simulink model "capsubot_Simulation_comparison_LandC"  (R2019a)
settings: Solver=ode45  StartTime=0.0  StopTime=16  FixedStep=.0001  MaxStep=.001  MinStep=.000001  RelTol=1e-3  EnableMultiTasking=on
values from neighbouring files (symbols this model uses):
  a1 = -a_stoke    [capsubot_dataperfectLuGree.m]
  a_c_desired_backward = [-a_all1' -a_all2']    [capsubot_dataperfectLuGree.m]
  a_u_desired = [a_all2' a_all1' a_all1' a_all2']    [capsubot_dataperfectLuGree.m]
  a_u_desired_backward = [-a_all2' -a_all1' -a_all1' -a_all2']    [capsubot_dataperfectLuGree.m]
  f_sm = data(8)    [capsubot_dataperfectLuGree.m]
  f_sM = 0.49    [capsubot_dataperfectLuGree.m]
  fv_Cap = data(9)    [capsubot_dataperfectLuGree.m]
  fv_IM = data(9)    [capsubot_dataperfectLuGree.m]
  g = 9.8    [capsubot_dataperfectLuGree.m]
  j = 30    [capsubot_dataperfectLuGree.m]
  k1 = 300    [capsubot_dataperfectLuGree.m]
  k2 = 100    [capsubot_dataperfectLuGree.m]
  m = data(2)    [capsubot_dataperfectLuGree.m]
  M = data(1)    [capsubot_dataperfectLuGree.m]
  m1 = data(2)    [capsubot_dataperfectLuGree.m]
  mu = data(3)    [capsubot_dataperfectLuGree.m]
  mu_1 = data(4)    [capsubot_dataperfectLuGree.m]
  mu_m = data(4)    [capsubot_dataperfectLuGree.m]
  sig_cap0 = data(8)    [capsubot_dataperfectLuGree.m]
  sig_cap1 = data(11)    [capsubot_dataperfectLuGree.m]
  sig_IM0 = data(8)    [capsubot_dataperfectLuGree.m]
  sig_IM1 = data(9)    [capsubot_dataperfectLuGree.m]
  tc = zeros(n,2)    [capsubot_dataperfectLuGree.m]
  tu = zeros(n,4)    [capsubot_dataperfectLuGree.m]
  z_cap = data(7)    [capsubot_dataperfectLuGree.m]
  z_IM = data(9)    [capsubot_dataperfectLuGree.m]
undefined symbols (not defined in the file or in its folder): profile, time_sim_individual_cum
libraries: fuzblock x2
(part 1 of 3)
settings Model: Creator=ERAS  LastModifiedBy=moham911
settings SolverCC: InitialStep=.001
settings DataIOCC: SaveFormat=Array  ReturnWorkspaceOutputs=off
settings OptimizationCC: ExpressionDepthLimit=2147483647  LifeSpan=inf
settings DebuggingCC: UnderspecifiedInitializationDetection=Classic  MergeDetectMultiDrivingBlocksExec=none  SolverPrmCheckMsg=warning  FcnCallInpInsideContextMsg=warning  StateNameClashWarn=warning  SFUnexpectedBacktrackingDiag=warning  SFNoUnconditionalDefaultTransitionDiag=warning  SFExecutionAtInitializationDiag=none  ArithmeticOperatorsInVariantConditions=warning
settings HardwareCC: ProdBitPerPointer=32  ProdBitPerSizeT=32  ProdBitPerPtrDiffT=32  ProdLargestAtomicFloat=None  ProdIntDivRoundTo=Undefined  ProdEndianess=Unspecified  ProdWordSize=32  ProdHWDeviceType=32-bit Generic
settings ModelReferenceCC: PropagateSignalLabelsOutOfModel=off
settings SFSimCC: SimUseLocalCustomCode=off
settings RTWCC: RTWUseLocalCustomCode=off
settings CodeAppCC: StateflowObjectComments=on
settings GRTTargetCC: TargetLangStandard=C89/C90 (ANSI)  GeneratePreprocessorConditionals=Disable all  CombineOutputUpdateFcns=off  GRTInterface=on
settings ConfigComp: CovMetricSettings=dw  CovHtmlReporting=on  CovSaveCumulativeToWorkspaceVar=on  CovSaveSingleToWorkspaceVar=on  CovExternalEMLEnable=off

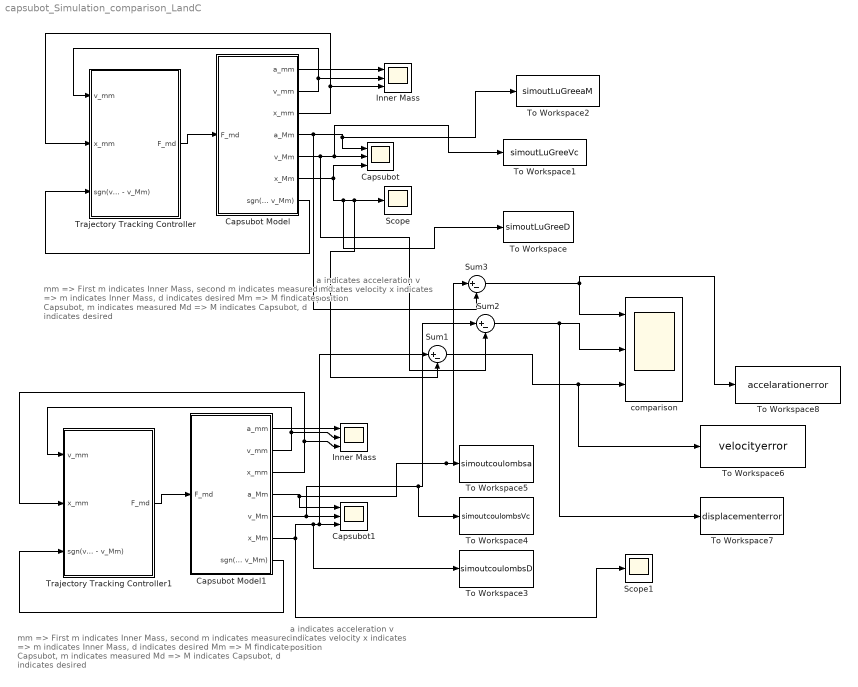
== system capsubot_Simulation_comparison_LandC ==
  note: a indicates acceleration
      | v indicates velocity
      | x indicates position
  note: mm => First m indicates Inner Mass, second m indicates measured
      | md => m indicates Inner Mass, d indicates desired
      | Mm => M findicates Capsubot, m indicates measured
      | Md => M indicates Capsubot, d indicates desired
  note: mm => First m indicates Inner Mass, second m indicates measured
      | md => m indicates Inner Mass, d indicates desired
      | Mm => M findicates Capsubot, m indicates measured
      | Md => M indicates Capsubot, d indicates desired
  note: a indicates acceleration
      | v indicates velocity
      | x indicates position
  " Capsubot Model" : Subsystem
  " Capsubot Model1" : Subsystem
  " Trajectory Tracking Controller" : Subsystem
  " Trajectory Tracking Controller1" : Subsystem
  Capsubot : Scope  NumInputPorts=3
  Capsubot1 : Scope  NumInputPorts=3
  Inner Mass : Scope  NumInputPorts=3
  "Inner Mass " : Scope  NumInputPorts=3
  Scope : Scope
  Scope1 : Scope
  Sum1 : Sum  Inputs=|+-
  Sum2 : Sum  Inputs=|+-
  Sum3 : Sum  Inputs=|+-
  To Workspace : ToWorkspace  VariableName=simoutLuGreeD  SaveFormat=Timeseries  SampleTime=-1
  To Workspace1 : ToWorkspace  VariableName=simoutLuGreeVc  SaveFormat=Timeseries  SampleTime=-1
  To Workspace2 : ToWorkspace  VariableName=simoutLuGreeaM  SaveFormat=Timeseries  SampleTime=-1
  To Workspace3 : ToWorkspace  VariableName=simoutcoulombsD  SaveFormat=Timeseries  SampleTime=-1
  To Workspace4 : ToWorkspace  VariableName=simoutcoulombsVc  SaveFormat=Timeseries  SampleTime=-1
  To Workspace5 : ToWorkspace  VariableName=simoutcoulombsa  SaveFormat=Timeseries  SampleTime=-1
  To Workspace6 : ToWorkspace  VariableName=velocityerror  SaveFormat=Timeseries  SampleTime=-1
  To Workspace7 : ToWorkspace  VariableName=displacementerror  SaveFormat=Timeseries  SampleTime=-1
  To Workspace8 : ToWorkspace  VariableName=accelarationerror  SaveFormat=Timeseries  SampleTime=-1
  "comparison " : Scope  NumInputPorts=3
  wires:
  " Capsubot Model"/2(v_mm) -> " Trajectory Tracking Controller"/1(v_mm), "Inner Mass "/2
  " Capsubot Model"/3(x_mm) -> " Trajectory Tracking Controller"/2(x_mm), "Inner Mass "/3
  " Capsubot Model"/1(a_mm) -> "Inner Mass "/1
  " Capsubot Model"/4(a_Mm) -> Sum3/2, To Workspace2/1, Capsubot/1
  " Capsubot Model"/5(v_Mm) -> Sum2/2, To Workspace1/1, Capsubot/2
  " Capsubot Model"/6(x_Mm) -> Capsubot/3, To Workspace/1, Sum1/2, Scope/1
  " Capsubot Model"/7(sgn(v_mm - v_Mm)) -> " Trajectory Tracking Controller"/3(sgn(v_mm - v_Mm))
  " Trajectory Tracking Controller"/1(F_md) -> " Capsubot Model"/1(F_md)
  " Capsubot Model1"/6(x_Mm) -> Scope1/1, To Workspace3/1, Sum1/1, Capsubot1/3
  " Capsubot Model1"/2(v_mm) -> Inner Mass/2, " Trajectory Tracking Controller1"/1(v_mm)
  " Capsubot Model1"/3(x_mm) -> " Trajectory Tracking Controller1"/2(x_mm), Inner Mass/3
  " Capsubot Model1"/4(a_Mm) -> Sum3/1, To Workspace5/1, Capsubot1/1
  " Capsubot Model1"/5(v_Mm) -> Capsubot1/2, Sum2/1, To Workspace4/1
  " Capsubot Model1"/1(a_mm) -> Inner Mass/1
  " Capsubot Model1"/7(sgn(v_mm - v_Mm)) -> " Trajectory Tracking Controller1"/3(sgn(v_mm - v_Mm))
  " Trajectory Tracking Controller1"/1(F_md) -> " Capsubot Model1"/1(F_md)
  Sum1/1 -> To Workspace6/1, "comparison "/3
  Sum2/1 -> To Workspace7/1, "comparison "/2
  Sum3/1 -> "comparison "/1, To Workspace8/1

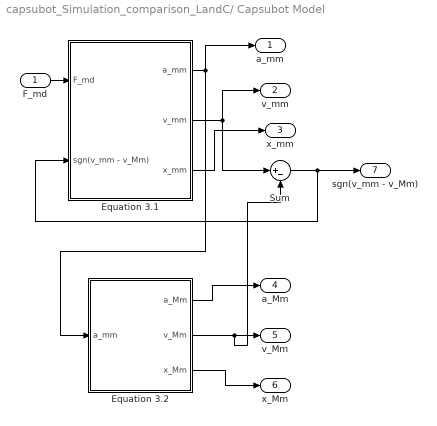
== system capsubot_Simulation_comparison_LandC/ Capsubot Model ==
  F_md : Inport
  Equation 3.1 : Subsystem
  Equation 3.2 : Subsystem
  Sum : Sum  Inputs=|+-
  a_mm : Outport
  v_mm : Outport  Port=2
  x_mm : Outport  Port=3
  a_Mm : Outport  Port=4
  v_Mm : Outport  Port=5
  x_Mm : Outport  Port=6
  sgn(v_mm - v_Mm) : Outport  Port=7
  wires:
  F_md/1 -> Equation 3.1/1(F_md)
  Equation 3.1/1(a_mm) -> a_mm/1, Equation 3.2/1(a_mm)
  Equation 3.1/2(v_mm) -> v_mm/1, Sum/1
  Equation 3.1/3(x_mm) -> x_mm/1
  Equation 3.2/1(a_Mm) -> a_Mm/1
  Equation 3.2/2(v_Mm) -> Sum/2, v_Mm/1
  Equation 3.2/3(x_Mm) -> x_Mm/1
  Sum/1 -> sgn(v_mm - v_Mm)/1, Equation 3.1/2(sgn(v_mm - v_Mm))

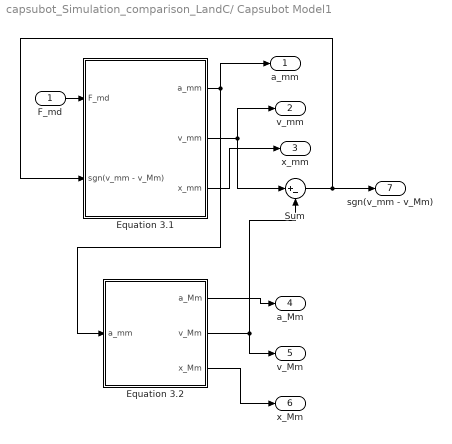
== system capsubot_Simulation_comparison_LandC/ Capsubot Model1 ==
  F_md : Inport
  Equation 3.1 : Subsystem
  Equation 3.2 : Subsystem
  Sum : Sum  Inputs=|+-
  a_mm : Outport
  v_mm : Outport  Port=2
  x_mm : Outport  Port=3
  a_Mm : Outport  Port=4
  v_Mm : Outport  Port=5
  x_Mm : Outport  Port=6
  sgn(v_mm - v_Mm) : Outport  Port=7
  wires:
  F_md/1 -> Equation 3.1/1(F_md)
  Equation 3.1/1(a_mm) -> a_mm/1, Equation 3.2/1(a_mm)
  Equation 3.1/2(v_mm) -> v_mm/1, Sum/1
  Equation 3.1/3(x_mm) -> x_mm/1
  Equation 3.2/1(a_Mm) -> a_Mm/1
  Equation 3.2/2(v_Mm) -> v_Mm/1, Sum/2
  Equation 3.2/3(x_Mm) -> x_Mm/1
  Sum/1 -> sgn(v_mm - v_Mm)/1, Equation 3.1/2(sgn(v_mm - v_Mm))

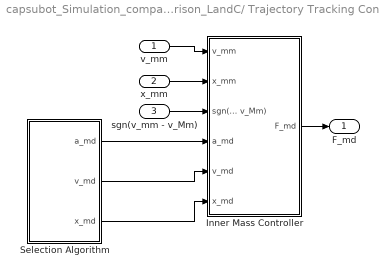
== system capsubot_Simulation_comparison_LandC/ Trajectory Tracking Controller ==
  v_mm : Inport
  x_mm : Inport  Port=2
  sgn(v_mm - v_Mm) : Inport  Port=3
  Inner Mass Controller : Subsystem
  Selection Algorithm : Subsystem
  F_md : Outport
  wires:
  Selection Algorithm/1(a_md) -> Inner Mass Controller/4(a_md)
  Selection Algorithm/3(x_md) -> Inner Mass Controller/6(x_md)
  sgn(v_mm - v_Mm)/1 -> Inner Mass Controller/3(sgn(v_mm - v_Mm))
  Selection Algorithm/2(v_md) -> Inner Mass Controller/5(v_md)
  Inner Mass Controller/1(F_md) -> F_md/1
  v_mm/1 -> Inner Mass Controller/1(v_mm)
  x_mm/1 -> Inner Mass Controller/2(x_mm)

== system capsubot_Simulation_comparison_LandC/ Trajectory Tracking Controller1 ==
  v_mm : Inport
  x_mm : Inport  Port=2
  sgn(v_mm - v_Mm) : Inport  Port=3
  Inner Mass Controller : Subsystem
  Selection Algorithm : Subsystem
  F_md : Outport
  wires:
  Selection Algorithm/1(a_md) -> Inner Mass Controller/4(a_md)
  Selection Algorithm/3(x_md) -> Inner Mass Controller/6(x_md)
  sgn(v_mm - v_Mm)/1 -> Inner Mass Controller/3(sgn(v_mm - v_Mm))
  Selection Algorithm/2(v_md) -> Inner Mass Controller/5(v_md)
  Inner Mass Controller/1(F_md) -> F_md/1
  v_mm/1 -> Inner Mass Controller/1(v_mm)
  x_mm/1 -> Inner Mass Controller/2(x_mm)

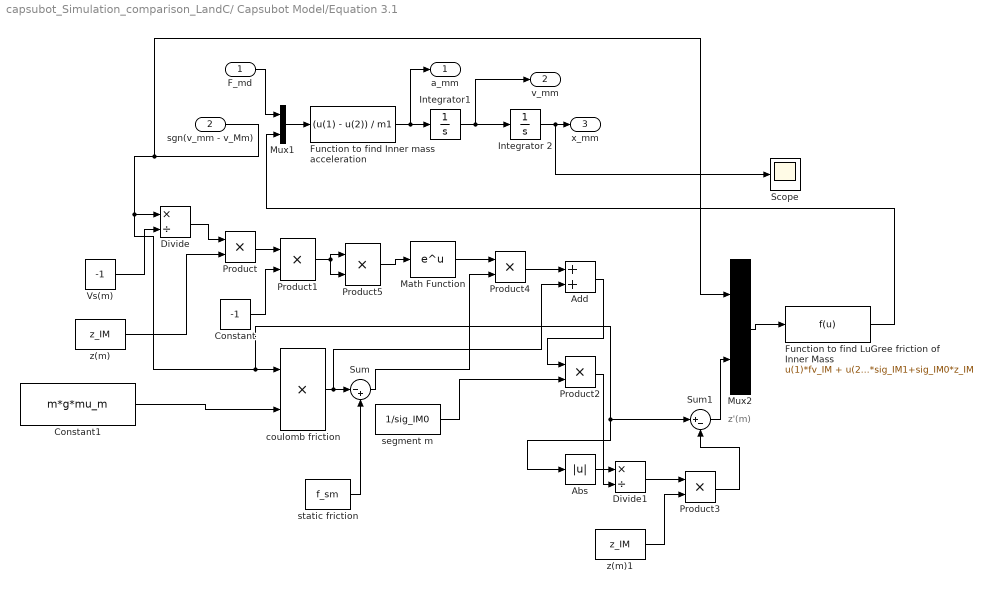
== system capsubot_Simulation_comparison_LandC/ Capsubot Model/Equation 3.1 ==
  note: z'(m)
  F_md : Inport
  sgn(v_mm - v_Mm) : Inport  Port=2
  Abs : Abs
  Add : Sum
  Constant : Constant  Value=-1
  Constant1 : Constant  Value=m*g*mu_m
  Divide : Product  Inputs=*/
  Divide1 : Product  Inputs=*/
  Function to find Inner mass acceleration : Fcn  Expr=(u(1) - u(2)) / m1
  "Function to find LuGree friction of Inner Mass " : Fcn  Expr=u(1)*fv_IM + u(2)*sig_IM1+sig_IM0*z_IM
  Integrator 2 : Integrator  InitialCondition=a1
  Integrator1 : Integrator
  Math Function : Math  SaturateOnIntegerOverflow=on
  Mux1 : Mux  Inputs=2
  Mux2 : Mux  Inputs=2
  Product{,1..5} (6 alike) : Product
  Scope : Scope
  Sum : Sum  Inputs=|-+
  Sum1 : Sum  Inputs=|+-
  Vs(m) : Constant  Value=-1
  "coulomb friction " : Product
  segment m : Constant  Value=1/sig_IM0
  "static friction " : Constant  Value=f_sm
  z(m) : Constant  Value=z_IM
  z(m)1 : Constant  Value=z_IM
  a_mm : Outport
  v_mm : Outport  Port=2
  x_mm : Outport  Port=3
  wires:
  "Function to find LuGree friction of Inner Mass "/1 -> Mux1/2
  Mux1/1 -> Function to find Inner mass acceleration/1
  F_md/1 -> Mux1/1
  Integrator1/1 -> v_mm/1, Integrator 2/1
  Integrator 2/1 -> Scope/1, x_mm/1
  Function to find Inner mass acceleration/1 -> a_mm/1, Integrator1/1
  segment m/1 -> Product2/2
  Product/1 -> Product1/1
  z(m)/1 -> Product/2
  Math Function/1 -> Product4/1
  Product4/1 -> Add/1
  Vs(m)/1 -> Divide/2
  "static friction "/1 -> Sum/2
  Sum/1 -> Product4/2
  Constant1/1 -> "coulomb friction "/2
  Constant/1 -> Product1/2
  Add/1 -> Product2/1
  "coulomb friction "/1 -> Add/2, Sum/1
  Divide/1 -> Product/1
  sgn(v_mm - v_Mm)/1 -> Mux2/1, Abs/1, Sum1/1, "coulomb friction "/1, Divide/1
  Abs/1 -> Divide1/1
  Product2/1 -> Divide1/2
  z(m)1/1 -> Product3/2
  Mux2/1 -> "Function to find LuGree friction of Inner Mass "/1
  Product5/1 -> Math Function/1
  Product1/1 -> Product5/2, Product5/1
  Divide1/1 -> Product3/1
  Product3/1 -> Sum1/2
  Sum1/1 -> Mux2/2

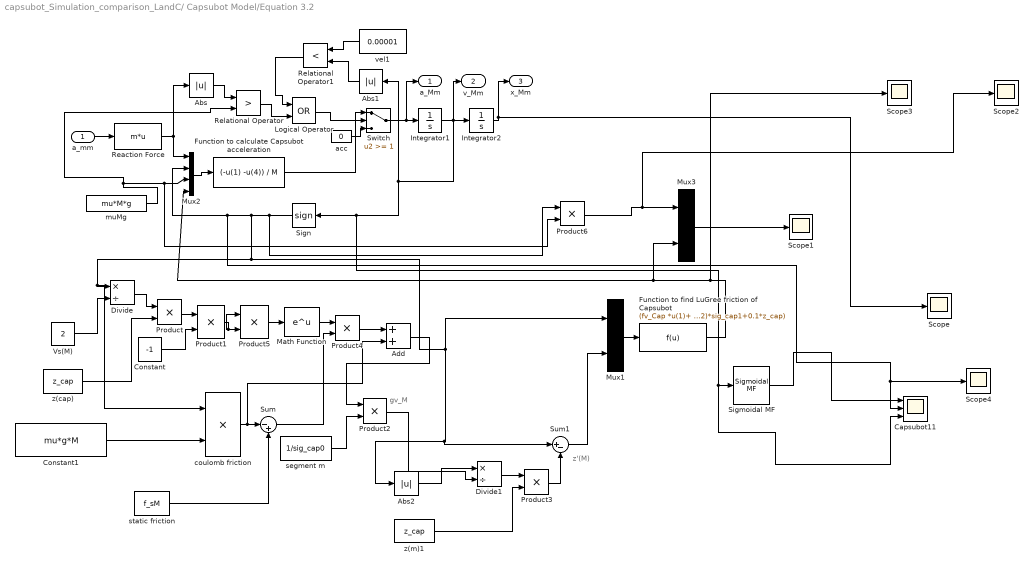
== system capsubot_Simulation_comparison_LandC/ Capsubot Model/Equation 3.2 ==
  note: gv_M
  note: z'(M)
  a_mm : Inport
  Abs : Abs
  Abs1 : Abs
  Abs2 : Abs
  Add : Sum
  Capsubot11 : Scope  NumInputPorts=3
  Constant : Constant  Value=-1
  Constant1 : Constant  Value=mu*g*M
  Divide : Product  Inputs=*/
  Divide1 : Product  Inputs=*/
  Function to calculate Capsubot acceleration : Fcn  Expr=(-u(1) -u(4)) / M
  "Function to find LuGree friction of Capsubot " : Fcn  Expr=(fv_Cap *u(1)+ u(2)*sig_cap1+0.1*z_cap)
  Integrator1 : Integrator
  Integrator2 : Integrator
  Logical Operator : Logic  Operator=OR  AllPortsSameDT=off  OutDataTypeStr=boolean
  Math Function : Math  SaturateOnIntegerOverflow=on
  Mux1 : Mux  Inputs=2
  Mux2 : Mux
  Mux3 : Mux  Inputs=2
  Product{,1..6} (7 alike) : Product
  Reaction Force : Fcn  Expr=m*u
  Relational Operator : RelationalOperator  Operator=>  OutDataTypeStr=boolean  RndMeth=Nearest
  Relational Operator1 : RelationalOperator  Operator=<  OutDataTypeStr=boolean  RndMeth=Nearest
  Scope{,1..4} (5 alike) : Scope
  Sigmoidal MF : fuzblock/Membership  Functions/Sigmoidal MF  a=1/1000  c=0
      settings: SourceProductName=Fuzzy Logic Toolbox  SourceProductBaseCode=FL
  Sign : Signum  ZeroCross=off
  Sum : Sum  Inputs=|-+
  Sum1 : Sum  Inputs=|+-
  Switch : Switch  Threshold=1
  Vs(M) : Constant  Value=2
  acc : Constant  Value=0
  "coulomb friction " : Product
  muMg : Constant  Value=mu*M*g
  segment m : Constant  Value=1/sig_cap0
  "static friction " : Constant  Value=f_sM
  vel1 : Constant  Value=0.00001
  z(cap) : Constant  Value=z_cap
  z(m)1 : Constant  Value=z_cap
  a_Mm : Outport
  v_Mm : Outport  Port=2
  x_Mm : Outport  Port=3
  wires:
  Mux2/1 -> Function to calculate Capsubot acceleration/1
  Abs/1 -> Relational Operator/1
  Function to calculate Capsubot acceleration/1 -> Switch/1
  acc/1 -> Switch/3
  Relational Operator/1 -> Logical Operator/2
  Logical Operator/1 -> Switch/2
  Relational Operator1/1 -> Logical Operator/1
  vel1/1 -> Relational Operator1/1
  Abs1/1 -> Relational Operator1/2
  Sign/1 -> Product6/1, Sum1/1, Abs2/1, Mux1/1, "coulomb friction "/1, Divide/1, Scope4/1, Capsubot11/2, Mux2/2
  muMg/1 -> Relational Operator/2, Product6/2, Mux2/3
  Reaction Force/1 -> Abs/1, Mux2/1
  a_mm/1 -> Reaction Force/1
  Switch/1 -> a_Mm/1, Integrator1/1
  "Function to find LuGree friction of Capsubot "/1 -> Scope3/1, Mux3/2, Mux2/4
  Vs(M)/1 -> Divide/2
  Product4/1 -> Add/1
  Product/1 -> Product1/1
  z(cap)/1 -> Product/2
  segment m/1 -> Product2/2
  Product2/1 -> Divide1/2
  Abs2/1 -> Divide1/1
  Sum/1 -> Product4/2
  "static friction "/1 -> Sum/2
  Constant/1 -> Product1/2
  "coulomb friction "/1 -> Add/2, Sum/1
  Divide/1 -> Product/1
  Integrator1/1 -> Integrator2/1, v_Mm/1, Capsubot11/3, Sigmoidal MF/1, Sign/1, Abs1/1
  Mux1/1 -> "Function to find LuGree friction of Capsubot "/1
  Math Function/1 -> Product4/1
  z(m)1/1 -> Product3/2
  Add/1 -> Product2/1
  Product1/1 -> Product5/1, Product5/2
  Product5/1 -> Math Function/1
  Constant1/1 -> "coulomb friction "/2
  Integrator2/1 -> Scope/1, x_Mm/1
  Divide1/1 -> Product3/1
  Product3/1 -> Sum1/2
  Sum1/1 -> Mux1/2
  Product6/1 -> Scope2/1, Mux3/1
  Mux3/1 -> Scope1/1
  Sigmoidal MF/1 -> Capsubot11/1

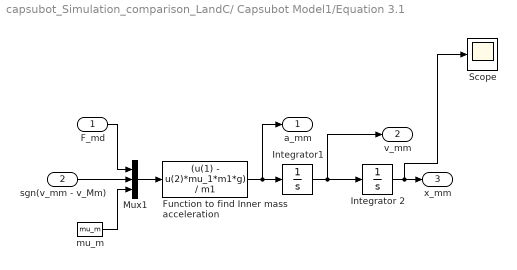
== system capsubot_Simulation_comparison_LandC/ Capsubot Model1/Equation 3.1 ==
  F_md : Inport
  sgn(v_mm - v_Mm) : Inport  Port=2
  Function to find Inner mass acceleration : Fcn  Expr=(u(1) - u(2)*mu_1*m1*g) / m1
  Integrator 2 : Integrator  InitialCondition=a1
  Integrator1 : Integrator
  Mux1 : Mux  Inputs=3
  Scope : Scope
  mu_m : Constant  Value=mu_m
  a_mm : Outport
  v_mm : Outport  Port=2
  x_mm : Outport  Port=3
  wires:
  mu_m/1 -> Mux1/3
  Mux1/1 -> Function to find Inner mass acceleration/1
  F_md/1 -> Mux1/1
  sgn(v_mm - v_Mm)/1 -> Mux1/2
  Integrator1/1 -> v_mm/1, Integrator 2/1
  Integrator 2/1 -> Scope/1, x_mm/1
  Function to find Inner mass acceleration/1 -> a_mm/1, Integrator1/1

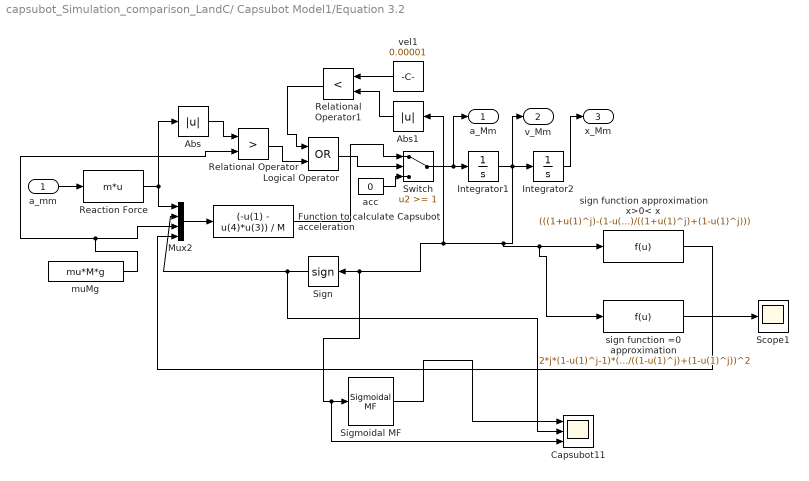
== system capsubot_Simulation_comparison_LandC/ Capsubot Model1/Equation 3.2 ==
  a_mm : Inport
  Abs : Abs
  Abs1 : Abs
  Capsubot11 : Scope  NumInputPorts=3
  Function to calculate Capsubot acceleration : Fcn  Expr=(-u(1) - u(4)*u(3)) / M
  Integrator1 : Integrator
  Integrator2 : Integrator
  Logical Operator : Logic  Operator=OR  AllPortsSameDT=off  OutDataTypeStr=boolean
  Mux2 : Mux
  Reaction Force : Fcn  Expr=m*u
  Relational Operator : RelationalOperator  Operator=>  OutDataTypeStr=boolean  RndMeth=Nearest
  Relational Operator1 : RelationalOperator  Operator=<  OutDataTypeStr=boolean  RndMeth=Nearest
  Scope1 : Scope
  Sigmoidal MF : fuzblock/Membership  Functions/Sigmoidal MF  a=1  c=0
      settings: SourceProductName=Fuzzy Logic Toolbox  SourceProductBaseCode=FL
  Sign : Signum  ZeroCross=off
  Switch : Switch  Threshold=1
  acc : Constant  Value=0
  muMg : Constant  Value=mu*M*g
  sign function approximation x>0< x : Fcn  Expr=(((1+u(1)^j)-(1-u(1)^j))/((1+u(1)^j)+(1-u(1)^j)))
  "sign function =0 approximation " : Fcn  Expr=2*j*(1-u(1)^j-1)*(1-u(1)^j)+(1-u(1)^j-1)*(1-u(1)^j)/((1-u(1)^j)+(1-u(1)^j))^2
  vel1 : Constant  Value=0.00001
  a_Mm : Outport
  v_Mm : Outport  Port=2
  x_Mm : Outport  Port=3
  wires:
  Mux2/1 -> Function to calculate Capsubot acceleration/1
  Abs/1 -> Relational Operator/1
  Function to calculate Capsubot acceleration/1 -> Switch/1
  acc/1 -> Switch/3
  Relational Operator/1 -> Logical Operator/2
  Logical Operator/1 -> Switch/2
  Relational Operator1/1 -> Logical Operator/1
  vel1/1 -> Relational Operator1/1
  Abs1/1 -> Relational Operator1/2
  Sign/1 -> Capsubot11/2, Mux2/2
  Integrator1/1 -> Integrator2/1, v_Mm/1, "sign function =0 approximation "/1, sign function approximation x>0< x/1, Capsubot11/3, Sigmoidal MF/1, Sign/1, Abs1/1
  muMg/1 -> Mux2/3, Relational Operator/2
  Reaction Force/1 -> Abs/1, Mux2/1
  a_mm/1 -> Reaction Force/1
  Switch/1 -> a_Mm/1, Integrator1/1
  Integrator2/1 -> x_Mm/1
  Sigmoidal MF/1 -> Capsubot11/1
  sign function approximation x>0< x/1 -> Mux2/4
  "sign function =0 approximation "/1 -> Scope1/1

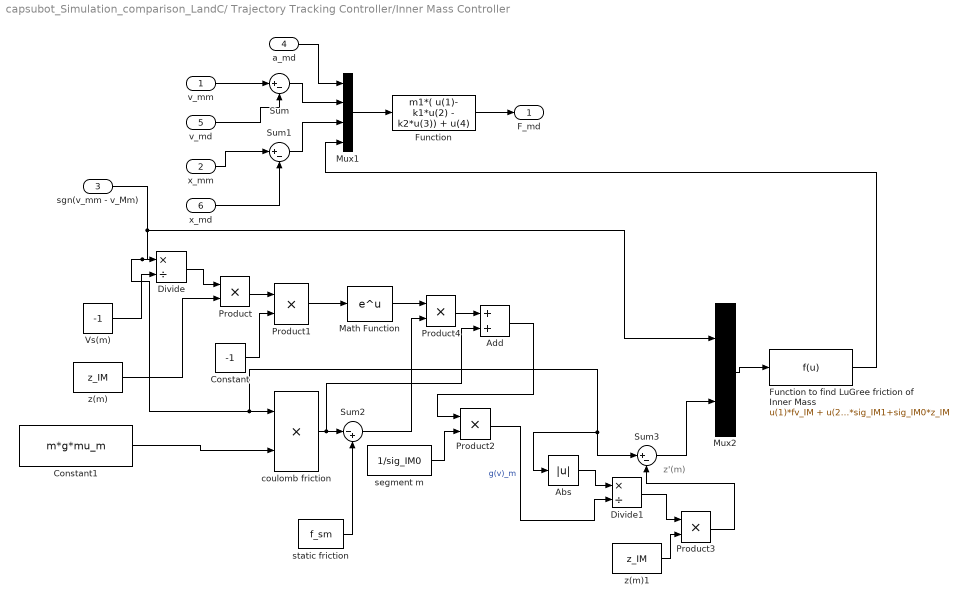
== system capsubot_Simulation_comparison_LandC/ Trajectory Tracking Controller/Inner Mass Controller ==
  note: z'(m)
  v_mm : Inport
  x_mm : Inport  Port=2
  sgn(v_mm - v_Mm) : Inport  Port=3
  a_md : Inport  Port=4
  v_md : Inport  Port=5
  x_md : Inport  Port=6
  Abs : Abs
  Add : Sum
  Constant : Constant  Value=-1
  Constant1 : Constant  Value=m*g*mu_m
  Divide : Product  Inputs=*/
  Divide1 : Product  Inputs=*/
  Function : Fcn  Expr=m1*( u(1)- k1*u(2) - k2*u(3)) + u(4)
  "Function to find LuGree friction of Inner Mass " : Fcn  Expr=u(1)*fv_IM + u(2)*sig_IM1+sig_IM0*z_IM
  Math Function : Math  SaturateOnIntegerOverflow=on
  Mux1 : Mux
  Mux2 : Mux  Inputs=2
  Product{,1..4} (5 alike) : Product
  Sum : Sum  Inputs=|+-
  Sum1 : Sum  Inputs=|+-
  Sum2 : Sum  Inputs=|-+
  Sum3 : Sum  Inputs=|+-
  Vs(m) : Constant  Value=-1
  "coulomb friction " : Product
  segment m : Constant  Value=1/sig_IM0
  "static friction " : Constant  Value=f_sm
  z(m) : Constant  Value=z_IM
  z(m)1 : Constant  Value=z_IM
  F_md : Outport
  wires:
  v_mm/1 -> Sum/1
  x_mm/1 -> Sum1/1
  Mux1/1 -> Function/1
  Function/1 -> F_md/1
  a_md/1 -> Mux1/1
  v_md/1 -> Sum/2
  x_md/1 -> Sum1/2
  Sum/1 -> Mux1/2
  Sum1/1 -> Mux1/3
  "Function to find LuGree friction of Inner Mass "/1 -> Mux1/4
  Constant1/1 -> "coulomb friction "/2
  Vs(m)/1 -> Divide/2
  Product4/1 -> Add/1
  Product/1 -> Product1/1
  z(m)/1 -> Product/2
  segment m/1 -> Product2/2
  Product2/1 -> Divide1/2  "g(v)_m"
  Abs/1 -> Divide1/1
  Sum2/1 -> Product4/2
  "static friction "/1 -> Sum2/2
  Constant/1 -> Product1/2
  "coulomb friction "/1 -> Add/2, Sum2/1
  Divide/1 -> Product/1
  sgn(v_mm - v_Mm)/1 -> Sum3/1, Abs/1, "coulomb friction "/1, Divide/1, Mux2/1
  Mux2/1 -> "Function to find LuGree friction of Inner Mass "/1
  Math Function/1 -> Product4/1
  Product1/1 -> Math Function/1
  z(m)1/1 -> Product3/2
  Add/1 -> Product2/1
  Divide1/1 -> Product3/1
  Product3/1 -> Sum3/2
  Sum3/1 -> Mux2/2

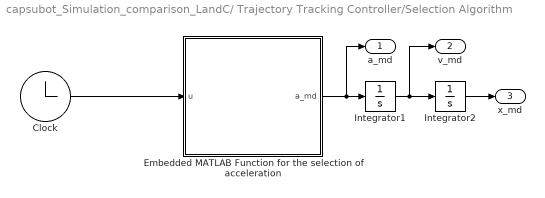
== system capsubot_Simulation_comparison_LandC/ Trajectory Tracking Controller/Selection Algorithm ==
  Clock : Clock
  "Embedded MATLAB Function for the selection of acceleration\t" : MATLAB Function  TreatAsAtomicUnit=on
  Integrator1 : Integrator
  Integrator2 : Integrator  InitialCondition=a1
  a_md : Outport
  v_md : Outport  Port=2
  x_md : Outport  Port=3
  wires:
  Integrator1/1 -> Integrator2/1, v_md/1
  Integrator2/1 -> x_md/1
  "Embedded MATLAB Function for the selection of acceleration\t"/1(a_md) -> a_md/1, Integrator1/1
  Clock/1 -> "Embedded MATLAB Function for the selection of acceleration\t"/1(u)

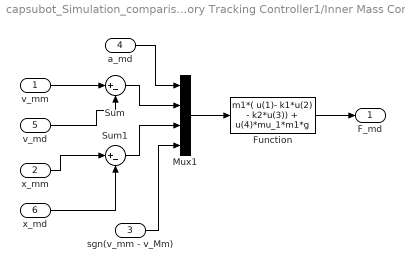
== system capsubot_Simulation_comparison_LandC/ Trajectory Tracking Controller1/Inner Mass Controller ==
  v_mm : Inport
  x_mm : Inport  Port=2
  sgn(v_mm - v_Mm) : Inport  Port=3
  a_md : Inport  Port=4
  v_md : Inport  Port=5
  x_md : Inport  Port=6
  Function : Fcn  Expr=m1*( u(1)- k1*u(2) - k2*u(3)) + u(4)*mu_1*m1*g
  Mux1 : Mux
  Sum : Sum  Inputs=|+-
  Sum1 : Sum  Inputs=|+-
  F_md : Outport
  wires:
  v_mm/1 -> Sum/1
  x_mm/1 -> Sum1/1
  Mux1/1 -> Function/1
  Function/1 -> F_md/1
  a_md/1 -> Mux1/1
  v_md/1 -> Sum/2
  x_md/1 -> Sum1/2
  Sum/1 -> Mux1/2
  Sum1/1 -> Mux1/3
  sgn(v_mm - v_Mm)/1 -> Mux1/4

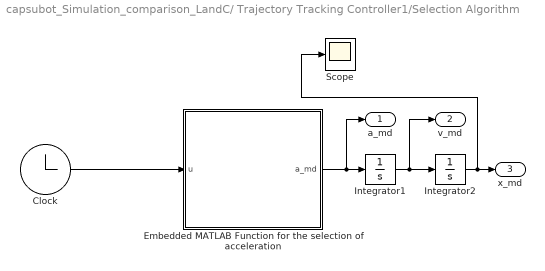
== system capsubot_Simulation_comparison_LandC/ Trajectory Tracking Controller1/Selection Algorithm ==
  Clock : Clock
  "Embedded MATLAB Function for the selection of acceleration\t" : MATLAB Function  TreatAsAtomicUnit=on
  Integrator1 : Integrator
  Integrator2 : Integrator  InitialCondition=a1
  Scope : Scope
  a_md : Outport
  v_md : Outport  Port=2
  x_md : Outport  Port=3
  wires:
  Integrator1/1 -> Integrator2/1, v_md/1
  Integrator2/1 -> Scope/1, x_md/1
  "Embedded MATLAB Function for the selection of acceleration\t"/1(a_md) -> a_md/1, Integrator1/1
  Clock/1 -> "Embedded MATLAB Function for the selection of acceleration\t"/1(u)
